simulink model "FlightGear"  (R2020b)
settings: Solver=VariableStepAuto  StartTime=0.0  StopTime=2  RelTol=1e-3
values from neighbouring files (symbols this model uses):
  A = [-0.0558 -0.9968 0.0802 0.0415; 0.5980 -0.1150 -0.0318 0; -3.0500 0.3880 -0.4650 0; 0 0.0805 1 0]    [AircraftPaper.m]
  B = [0.0729 0; -4.7500 0.00775; 0.153 0.143; 0 0]    [AircraftPaper.m]
  C = [1 0 0 0; 0 0 0 1]    [AircraftPaper.m]
  D = [0 0; 0 0]    [AircraftPaper.m]
  F = inversa(1:4)    [AircraftPaper.m]
  Kc = lqr(A,B,Q,R)    [AircraftPaper.m]
  N = inversa(5:6)    [AircraftPaper.m]
  x0 = [pi/6 0 0 pi/4]    [AircraftPaper.m]
undefined symbols (not defined in the file or in its folder): Earth, WGS84
libraries: cstblocks x3, aerolibutil x2, aerolibfltsims x2, simulink_extras x2, aerolibtransform2 x1, vrlib x1
settings Model: Creator=leobartowski  LastModifiedBy=leobartowski

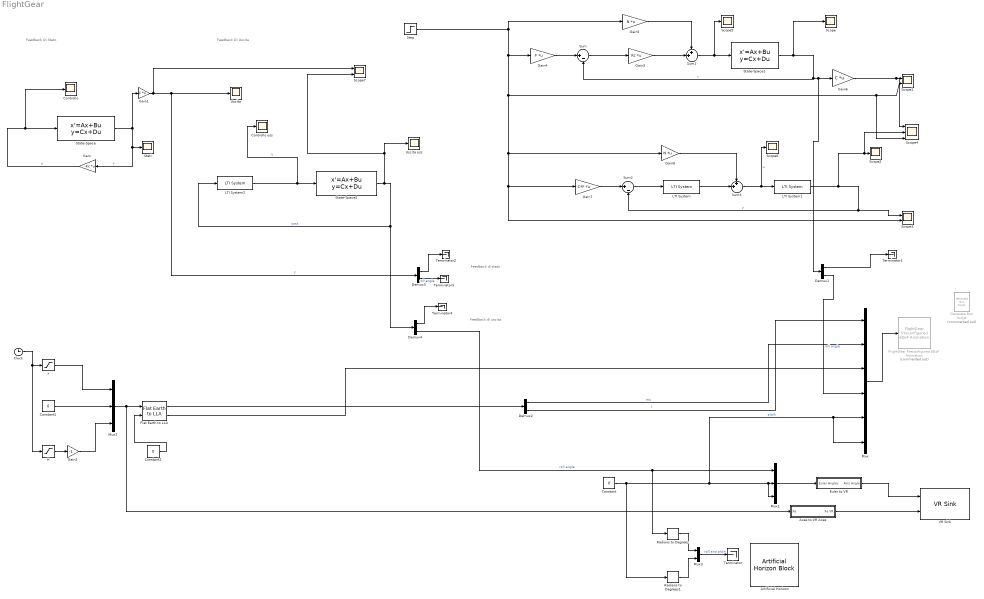
== system FlightGear ==
  note: Feedback di stato
  note: Feedback Di Uscita
  note: Feedback Di Stato
  note: Feedback di uscita
  Artificial Horizon : ArtificialHorizonBlock  LabelPosition=Bottom
  Axes to VR Axes : Subsystem
  Clock : Clock
  Constant : Constant  Value=0
  Constant1 : Constant  Value=0
  Constant2 : Constant  Value=0
  Controllo : Scope
  Controllo oss : Scope
  Demux{1..4} (4 alike) : Demux  Outputs=2
  Euler to VR : Subsystem
  Flat Earth to LLA : aerolibtransform2/Flat Earth to LLA  units=Metric (MKS)  ptype=Earth (WGS84)  F=1/298.257223563  R=6378137  refPosPort=off  LL0=[0 10]  psi=0
  FlightGear Preconfigured 6DoF Animation : aerolibfltsims/FlightGear Preconfigured 6DoF Animation  Commented=on  xFlightGearVersion=v2019.1  DestinationIpAddress=127.0.0.1  DestinationPort=5502  SampleTime=1/30  packetVersion=24
  Gain : Gain  Gain=-Kc  Multiplication=Matrix(K*u)
  Gain1 : Gain  Gain=C  Multiplication=Matrix(K*u)
  Gain2 : Gain  Gain=-1
  Gain3 : Gain  Gain=Kc  Multiplication=Matrix(K*u)
  Gain4 : Gain  Gain=F  Multiplication=Matrix(K*u)
  Gain5 : Gain  Gain=N  Multiplication=Matrix(K*u)
  Gain6 : Gain  Gain=C  Multiplication=Matrix(K*u)
  Gain7 : Gain  Gain=C*F  Multiplication=Matrix(K*u)
  Gain8 : Gain  Gain=N  Multiplication=Matrix(K*u)
  Generate Run Script : aerolibfltsims/Generate Run Script  Commented=on  Architecture=Mac  dataFlow=Send  GeometryModelName=HL20  AirportId=KSFO  RunwayId=10L  InitialAltitude=7224  InitialHeading=113  OffsetDistance=4.72  OffsetAzimuth=0  InstallScenery=on  DisableShaders=on  OriginAddress=127.0.0.1  DestinationPort=5502  OriginPort=5505  LocalAddress=127.0.0.1  OutputFileName=runfg.bat  FlightGearBaseDirectory=/Applications/FlightGear.app
  H : Saturate
  LTI System : cstblocks/LTI System  sys=Kset  IC=[]
  LTI System1 : cstblocks/LTI System  sys=Ps  IC=x0
  LTI System2 : cstblocks/LTI System  sys=K  IC=[]
  Mux : Mux  Inputs=6
  Mux1 : Mux  Inputs=3
  Mux2 : Mux  Inputs=3
  Mux3 : Mux  Inputs=2
  Radians to Degrees : simulink_extras/Transformations/Radians to Degrees
  Radians to Degrees1 : simulink_extras/Transformations/Radians to Degrees
  Scope{,2,5..6} (4 alike) : Scope
  Scope1 : Scope  NumInputPorts=2
  Scope3 : Scope  NumInputPorts=2
  Scope4 : Scope  NumInputPorts=3
  Scope7 : Scope  NumInputPorts=2
  State-Space : StateSpace  A=A  B=B  C=eye(4)  D=zeros(4,2)  InitialCondition=x0
  State-Space1 : StateSpace  A=A  B=B  C=eye(4)  D=zeros(4,2)  InitialCondition=x0
  State-Space2 : StateSpace  A=A  B=B  C=C  D=D  InitialCondition=x0
  Stati : Scope
  Step : Step  After=pi/4  SampleTime=3
  Sum : Sum  Inputs=|+-
  Sum1 : Sum  Inputs=++|
  Sum2 : Sum  Inputs=|+-
  Sum3 : Sum  Inputs=++|
  Terminator{,1..4} (5 alike) : Terminator
  Uscita : Scope
  Uscita oss : Scope
  VR Sink : vrlib/VR Sink  InstantiateOnLoad=on  SampleTime=0.005  ViewEnable=on  RemoteChange=off  RemoteView=off  FieldsWritten=HL20.rotation.4.1.1.double#HL20.translation.3.1.1.double  WorldFileName=world2.wrl  WorldDescription=Esame MFC  AutoView=on  VideoDimensions=[]  AllowVariableSize=off  FigureProperties="{'Position', 'Name', 'Viewpoint', 'CameraBound', 'CameraDirection', 'CameraPosition', 'CameraUpVector', 'ZoomFactor', 'Antialiasing', 'Headlight', 'Lighting', 'NavPanel', 'Sound', 'StatusBar', 'Stereo3D', 'Stereo3DCameraOffset', 'Stereo3DHIT', 'ToolBar', 'Textures', 'Transparency', 'Triad', 'Wireframe', 'NavZones', 'NavMode', 'NavSpeed', 'CaptureFileFormat', 'CaptureFileName', 'Record2DCompressMethod', 'Record2DCompressQuality', 'Record2D', 'Record2DFileName', 'Record2DFPS'; [-1.7250000000000000e+03   1.0300000000000000e+02   5.4400000000000000e+02   5.2700000000000000e+02], 'Esame MFC', 'Fixed Position', 'on', [0.0000000000000000e+00   0.0000000000000000e+00  -1.0000000000000000e+00], [0.0000000000000000e+00   0.0000000000000000e+00   7.0000000000000000e+01], [0.0000000000000000e+00   1.0000000000000000e+00   0.0000000000000000e+00], [1.0000000000000000e+00], 'on', 'on', 'on', 'halfbar', 'on', 'on', 'off', [1.0000000149011612e-01], [0.0000000000000000e+00], 'on', 'on', 'on', 'none', 'off', 'off', 'fly', 'normal', 'tif', '%f_anim_%n.tif', 'auto', [7.5000000000000000e+01], 'off', '%f_anim_%n.avi', 'auto'}"
  x : Saturate
  wires:
  Euler to VR/1(Axis Angle) -> VR Sink/1
  Axes to VR Axes/1(Xe VR) -> VR Sink/2
  Mux/1 -> FlightGear Preconfigured 6DoF Animation/1
  Clock/1 -> H/1, x/1
  x/1 -> Mux2/1
  Constant1/1 -> Mux2/2
  H/1 -> Gain2/1
  Gain2/1 -> Mux2/3
  Mux2/1 -> Axes to VR Axes/1(Xe), Flat Earth to LLA/1
  Constant2/1 -> Flat Earth to LLA/2
  Flat Earth to LLA/1 -> Demux2/1
  Demux2/2 -> Mux/1  "l"
  Demux2/1 -> Mux/2  "mu"
  Flat Earth to LLA/2 -> Mux/3
  Constant/1 -> Radians to Degrees1/1, Mux/6, Mux/5, Mux1/3, Mux1/2  "pitch"
  Mux1/1 -> Euler to VR/1(Euler Angles)
  Sum/1 -> Gain3/1
  Gain6/1 -> Scope4/1, Scope1/1
  Sum2/1 -> LTI System/1
  Gain5/1 -> Sum1/1
  Gain4/1 -> Sum/1
  Sum1/1 -> Scope5/1, State-Space1/1
  LTI System/1 -> Sum3/2
  Gain3/1 -> Sum1/2
  LTI System1/1 -> Scope4/2, Scope2/1, Scope3/1, Sum2/2  "y"
  State-Space1/1 -> Scope/1, Sum/2, Demux1/1, Gain6/1  "x"
  Sum3/1 -> LTI System1/1, Scope6/1  "u"
  Gain8/1 -> Sum3/1
  Step/1 -> Scope3/2, Gain7/1, Gain8/1, Scope4/3, Scope1/2, Gain4/1, Gain5/1
  Gain7/1 -> Sum2/1
  Demux1/2 -> Mux/4  "roll angle"
  Demux1/1 -> Terminator1/1
  State-Space/1 -> Gain1/1, Gain/1, Stati/1  "x"
  State-Space2/1 -> Demux4/1, LTI System2/1, Scope7/2, Uscita oss/1  "yoss"
  Gain/1 -> Controllo/1, State-Space/1  "u"
  Gain1/1 -> Scope7/1, Uscita/1, Demux3/1  "y"
  LTI System2/1 -> Controllo oss/1, State-Space2/1  "u"
  Demux3/1 -> Terminator2/1
  Demux3/2 -> Terminator3/1  "roll angle"
  Demux4/1 -> Terminator4/1
  Demux4/2 -> Radians to Degrees/1, Mux1/1  "roll angle"
  Mux3/1 -> Terminator/1  "roll and pitch"
  Radians to Degrees/1 -> Mux3/1
  Radians to Degrees1/1 -> Mux3/2

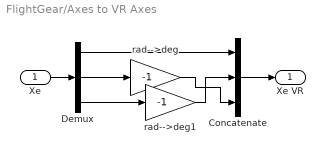
== system FlightGear/Axes to VR Axes ==
  Xe : Inport
  Concatenate : Concatenate  NumInputs=3
  Demux : Demux  Outputs=3
      settings: DisplayOption=none
  rad-->deg : Gain  Gain=-1  SaturateOnIntegerOverflow=on  OutDataTypeStr=Inherit: Same as input  ParamDataTypeStr=Inherit: Same as input
  rad-->deg1 : Gain  Gain=-1  SaturateOnIntegerOverflow=on  OutDataTypeStr=Inherit: Same as input  ParamDataTypeStr=Inherit: Same as input
  Xe VR : Outport  VectorParamsAs1DForOutWhenUnconnected=off
  wires:
  Xe/1 -> Demux/1
  Demux/1 -> Concatenate/1
  Demux/2 -> rad-->deg/1
  Demux/3 -> rad-->deg1/1
  Concatenate/1 -> Xe VR/1
  rad-->deg1/1 -> Concatenate/2
  rad-->deg/1 -> Concatenate/3

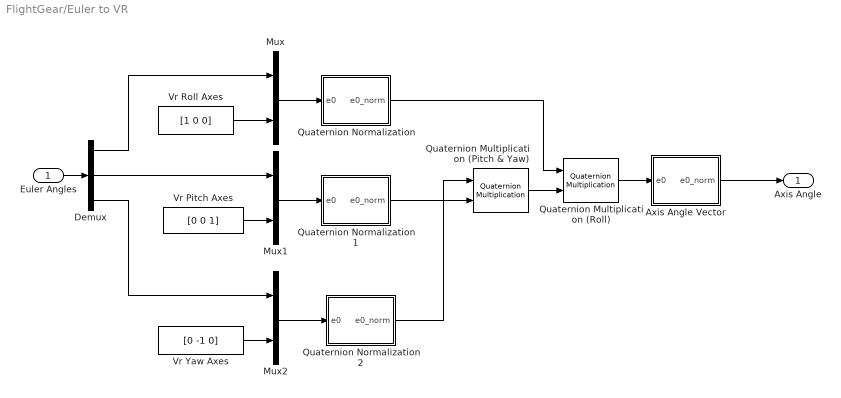
== system FlightGear/Euler to VR ==
  Euler Angles : Inport
  Axis Angle Vector : Subsystem
  Demux : Demux  Outputs=3
      settings: DisplayOption=none
  Mux : Mux  Inputs=2
  Mux1 : Mux  Inputs=2
  Mux2 : Mux  Inputs=2
  Quaternion Multiplication (Pitch & Yaw) : aerolibutil/Quaternion Multiplication
  Quaternion Multiplication (Roll) : aerolibutil/Quaternion Multiplication
  Quaternion Normalization : Subsystem
  Quaternion Normalization1 : Subsystem
  Quaternion Normalization2 : Subsystem
  Vr Pitch Axes : Constant  Value=[0 0 1]
  Vr Roll Axes : Constant  Value=[1 0 0]
  Vr Yaw Axes : Constant  Value=[0 -1 0]
  Axis Angle : Outport  VectorParamsAs1DForOutWhenUnconnected=off
  wires:
  Quaternion Multiplication (Roll)/1 -> Axis Angle Vector/1(e0)
  Quaternion Multiplication (Pitch & Yaw)/1 -> Quaternion Multiplication (Roll)/2
  Axis Angle Vector/1(e0_norm) -> Axis Angle/1
  Quaternion Normalization/1(e0_norm) -> Quaternion Multiplication (Roll)/1
  Quaternion Normalization2/1(e0_norm) -> Quaternion Multiplication (Pitch & Yaw)/1
  Quaternion Normalization1/1(e0_norm) -> Quaternion Multiplication (Pitch & Yaw)/2
  Mux2/1 -> Quaternion Normalization2/1(e0)
  Mux1/1 -> Quaternion Normalization1/1(e0)
  Mux/1 -> Quaternion Normalization/1(e0)
  Demux/3 -> Mux2/1
  Vr Yaw Axes/1 -> Mux2/2
  Demux/2 -> Mux1/1
  Vr Pitch Axes/1 -> Mux1/2
  Demux/1 -> Mux/1
  Vr Roll Axes/1 -> Mux/2
  Euler Angles/1 -> Demux/1

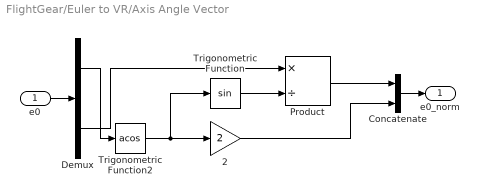
== system FlightGear/Euler to VR/Axis Angle Vector ==
  e0 : Inport
  2 : Gain  Gain=2  SaturateOnIntegerOverflow=on  OutDataTypeStr=Inherit: Same as input  ParamDataTypeStr=Inherit: Same as input
  Concatenate : Concatenate
  Demux : Demux  Outputs=[1 3 ]
      settings: DisplayOption=none
  Product : Product  Inputs=*/  InputSameDT=on  SaturateOnIntegerOverflow=on  OutDataTypeStr=Inherit: Same as first input
  Trigonometric Function : Trigonometry
  Trigonometric Function2 : Trigonometry  Operator=acos
  e0_norm : Outport  VectorParamsAs1DForOutWhenUnconnected=off
  wires:
  Demux/1 -> Trigonometric Function2/1
  Demux/2 -> Product/1
  Concatenate/1 -> e0_norm/1
  Product/1 -> Concatenate/1
  2/1 -> Concatenate/2
  Trigonometric Function/1 -> Product/2
  Trigonometric Function2/1 -> Trigonometric Function/1, 2/1
  e0/1 -> Demux/1

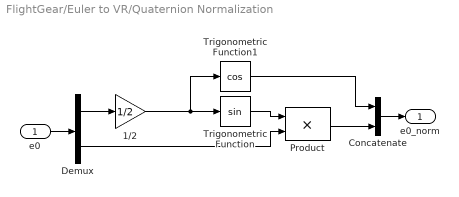
== system FlightGear/Euler to VR/Quaternion Normalization ==
  e0 : Inport
  1/2 : Gain  Gain=1/2  SaturateOnIntegerOverflow=on  OutDataTypeStr=Inherit: Same as input  ParamDataTypeStr=Inherit: Same as input
  Concatenate : Concatenate
  Demux : Demux  Outputs=[1 3]
      settings: DisplayOption=none
  Product : Product  InputSameDT=on  SaturateOnIntegerOverflow=on  OutDataTypeStr=Inherit: Same as first input
  Trigonometric Function : Trigonometry
  Trigonometric Function1 : Trigonometry  Operator=cos
  e0_norm : Outport  VectorParamsAs1DForOutWhenUnconnected=off
  wires:
  Trigonometric Function1/1 -> Concatenate/1
  Demux/2 -> Product/2
  Demux/1 -> 1/2/1
  Concatenate/1 -> e0_norm/1
  Product/1 -> Concatenate/2
  Trigonometric Function/1 -> Product/1
  1/2/1 -> Trigonometric Function1/1, Trigonometric Function/1
  e0/1 -> Demux/1

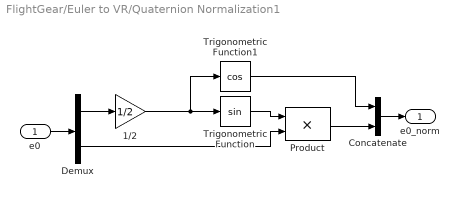
== system FlightGear/Euler to VR/Quaternion Normalization1 ==
  e0 : Inport
  1/2 : Gain  Gain=1/2  SaturateOnIntegerOverflow=on  OutDataTypeStr=Inherit: Same as input  ParamDataTypeStr=Inherit: Same as input
  Concatenate : Concatenate
  Demux : Demux  Outputs=[1 3]
      settings: DisplayOption=none
  Product : Product  InputSameDT=on  SaturateOnIntegerOverflow=on  OutDataTypeStr=Inherit: Same as first input
  Trigonometric Function : Trigonometry
  Trigonometric Function1 : Trigonometry  Operator=cos
  e0_norm : Outport  VectorParamsAs1DForOutWhenUnconnected=off
  wires:
  e0/1 -> Demux/1
  1/2/1 -> Trigonometric Function/1, Trigonometric Function1/1
  Trigonometric Function/1 -> Product/1
  Product/1 -> Concatenate/2
  Concatenate/1 -> e0_norm/1
  Demux/1 -> 1/2/1
  Demux/2 -> Product/2
  Trigonometric Function1/1 -> Concatenate/1

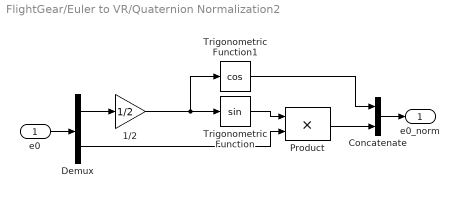
== system FlightGear/Euler to VR/Quaternion Normalization2 ==
  e0 : Inport
  1/2 : Gain  Gain=1/2  SaturateOnIntegerOverflow=on  OutDataTypeStr=Inherit: Same as input  ParamDataTypeStr=Inherit: Same as input
  Concatenate : Concatenate
  Demux : Demux  Outputs=[1 3]
      settings: DisplayOption=none
  Product : Product  InputSameDT=on  SaturateOnIntegerOverflow=on  OutDataTypeStr=Inherit: Same as first input
  Trigonometric Function : Trigonometry
  Trigonometric Function1 : Trigonometry  Operator=cos
  e0_norm : Outport  VectorParamsAs1DForOutWhenUnconnected=off
  wires:
  Trigonometric Function1/1 -> Concatenate/1
  Demux/2 -> Product/2
  Demux/1 -> 1/2/1
  Concatenate/1 -> e0_norm/1
  Product/1 -> Concatenate/2
  Trigonometric Function/1 -> Product/1
  1/2/1 -> Trigonometric Function1/1, Trigonometric Function/1
  e0/1 -> Demux/1
